simulink model "Solar_Seguidor_V2"  (R2021b)
settings: Solver=ode1  StartTime=0.0  StopTime=10  FixedStep=25e-6  RelTol=1e-3
PostLoadFcn:
  | %clc; clear all; close all;
  | %%%%%%%%%%%%%%%%%%%%%%%%%%%%%%%%%%%%%%%%%%%%%%%%
  | %%%%%%%%% Solar seguidor de rede %%%%%%%%%%
  | %%%%%%%%%%%%%%%%%%%%%%%%%%%%%%%%%%%%%%%%%%%%%%%%
  | %%%% Nominal Parameters %%%%
  | Pnom = 16e3;                                         % Potencia Nominal
  | Vnom_rms = 210;                                    % V linha rms
  | Vnom_peak = sqrt(2/3)*Vnom_rms;                     % V fase pico
  | FP_min = 1;                                       % Para suporte de reativo
  | Snom = Pnom/FP_min;                                 % Potencia aparente
  | Irms = Pnom/(sqrt(3)*Vnom_rms);                     % Ig rms
  | Inom_peak = Irms*sqrt(2);                           % Ig pico
  | Zbase = Vnom_peak/Inom_peak;                        % Impedancia Base
  | f = 60;                                             % Freq nominal
  | wnom = 2*pi*60;                                     % Freq Ang. nominal
  | m = 0.805;                                            % Indice mod nominal
  | Vdc = 2*(Vnom_peak/m);                              % Vcc
  | Vdc_2 = Vdc/2;                                      % Metade Vcc
  | Kconv = Zbase;                                      % Ganho conversor
  | %%%% Transformer %%%%
  | S_trafo = 250e3;                                      % transformer apparent power
  | Vrms_high = 400;                                   % transformer secondary voltage - Wye connection
  | Vrms_low = 210;                                   % transformer primary voltage - Delta connection
  | N = Vrms_high/Vrms_low;                             % transformation relationship
  | X_pu_trafo = 0.03;                                 % transformer p.u. reactance
  | Zb_trafo_high = ((Vrms_high)^2)/S_trafo;            % secondary base impedance
  | Zb_trafo = ((Vnom_rms)^2)/S_trafo;                  % primary base impedance
  | L_trafo = (X_pu_trafo*Zb_trafo)/wnom;               % primary inductance
  | %%%% LCL Filter Project %%%%
  | fsw = 105*60;%105*60;                                         % switching frequency
  | ripple = 0.05;                                       % current ripple
  | L1 = Vdc/(6*ripple*Inom_peak*fsw);                  % inductor L1
  |  RL1 = 0.005;                                        % L1 resistance
  |  Cbase = 1/(wnom*Kconv);                             % base capacitance
  |  Cf = 0.05*Cbase;                                    % filter capacitor
  | % Calculo do filtro
  | Sbase = 16e3;
  | %Sbase = 200e3*1.12;
  | V_LL = 210;
  | V_LG = 210/sqrt(3);
  | Vbase = V_LG*sqrt(2);
  | Ibase = (Sbase*sqrt(2))/(V_LG*3)*sqrt(3/2);
  | Zbase = (V_LL^2)/Sbase;
  | Rbase = Zbase;
  | Xbase = Zbase;
  | Lbase = Xbase/(2*pi*60);
  | Cbase = 1/(Xbase*2*pi*60);
  | w = 2*pi*60;
  | Q = 70;
  | Lf = 0.15*Lbase;
  | Cf = 0.05*Cbase;
  | fc = 1/(2*pi*sqrt(Lf*Cf));
  | R = (w*Lf)/Q;
  | Lf = L1;
  | R = RL1;
  | ka=0.2;                                             % attenuation factor
  | L2 = (sqrt(1/(ka^2))+1)/(Cf*((2*pi*fsw)^2));        % inductor L2
  | RL2 = 0.005;                                        % L2 resistance
  | w_res = sqrt((L1+L2+L_trafo)/(L1*L2*Cf));           % resonant angular frequency
  | f_res = w_res/(2*pi);                               % resonant frequency
  | Rf = 1/(3*w_res*Cf);                                % filter capacitor resistance
  | %%%%%%%%%%%%%%%%%%%%%%%%
  | %%%% Control Design %%%%
  | %%%%%%%%%%%%%%%%%%%%%%%%
  | %%%% Power Control %%%%
  | Ron = 0.0001;
  | tau_i = 0.5e-3;                                       % tempo de resposta
  | kp_current = (Lf+L_trafo)/tau_i;
  | ki_current = (R+Ron)/tau_i;
  | decouple = (wnom*Lf);
  | kp_current_pu = kp_current/Kconv;                  % Adaptando para pu
  | ki_current_pu = ki_current/Kconv;
  | decouple_pu = (wnom*Lf+(R+Ron))/Kconv;
  | %%%% Dc Link Control %%%%
  | Iext = Pnom/Vdc;
  | Kcc = Vdc/Iext;
  | Sbase = 16e3;
  | C_cc_proj = (Sbase/(2*pi*60*Vdc*Vdc*0.05));
  | 
  | % Controle de tensao
  | a = 3;
  | kp_dc = (C_cc_proj)/(2*a*tau_i);
  | ti_dc = (a^2)*tau_i;
  | ki_dc = kp_dc/ti_dc;
  | kp_dc_pu = (Kcc*C_cc_proj)/(2*a*tau_i);
  | ki_dc_pu = kp_dc_pu/ti_dc;
  | 
  | Ts =25e-6;
  | 
  | 
  |  Ts_Control=2*Ts;Ts_Power=Ts;
InitFcn:
  | %clc; clear all; close all;
  | %%%%%%%%%%%%%%%%%%%%%%%%%%%%%%%%%%%%%%%%%%%%%%%%
  | %%%%%%%%% Solar seguidor de rede %%%%%%%%%%
  | %%%%%%%%%%%%%%%%%%%%%%%%%%%%%%%%%%%%%%%%%%%%%%%%
  | %%%% Nominal Parameters %%%%
  | Pnom = 16e3;                                         % Potencia Nominal
  | Vnom_rms = 210;                                    % V linha rms
  | Vnom_peak = sqrt(2/3)*Vnom_rms;                     % V fase pico
  | FP_min = 1;                                       % Para suporte de reativo
  | Snom = Pnom/FP_min;                                 % Potencia aparente
  | Irms = Pnom/(sqrt(3)*Vnom_rms);                     % Ig rms
  | Inom_peak = Irms*sqrt(2);                           % Ig pico
  | Zbase = Vnom_peak/Inom_peak;                        % Impedancia Base
  | f = 60;                                             % Freq nominal
  | wnom = 2*pi*60;                                     % Freq Ang. nominal
  | m = 0.805;                                            % Indice mod nominal
  | Vdc = 2*(Vnom_peak/m);                              % Vcc
  | Vdc_2 = Vdc/2;                                      % Metade Vcc
  | Kconv = Zbase;                                      % Ganho conversor
  | %%%% Transformer %%%%
  | S_trafo = 250e3;                                      % transformer apparent power
  | Vrms_high = 400;                                   % transformer secondary voltage - Wye connection
  | Vrms_low = 210;                                   % transformer primary voltage - Delta connection
  | N = Vrms_high/Vrms_low;                             % transformation relationship
  | X_pu_trafo = 0.03;                                 % transformer p.u. reactance
  | Zb_trafo_high = ((Vrms_high)^2)/S_trafo;            % secondary base impedance
  | Zb_trafo = ((Vnom_rms)^2)/S_trafo;                  % primary base impedance
  | L_trafo = (X_pu_trafo*Zb_trafo)/wnom;               % primary inductance
  | %%%% LCL Filter Project %%%%
  | fsw = 105*60;%105*60;                                         % switching frequency
  | ripple = 0.05;                                       % current ripple
  | L1 = Vdc/(6*ripple*Inom_peak*fsw);                  % inductor L1
  |  RL1 = 0.005;                                        % L1 resistance
  |  Cbase = 1/(wnom*Kconv);                             % base capacitance
  |  Cf = 0.05*Cbase;                                    % filter capacitor
  | % Calculo do filtro
  | Sbase = 16e3;
  | %Sbase = 200e3*1.12;
  | V_LL = 210;
  | V_LG = 210/sqrt(3);
  | Vbase = V_LG*sqrt(2);
  | Ibase = (Sbase*sqrt(2))/(V_LG*3)*sqrt(3/2);
  | Zbase = (V_LL^2)/Sbase;
  | Rbase = Zbase;
  | Xbase = Zbase;
  | Lbase = Xbase/(2*pi*60);
  | Cbase = 1/(Xbase*2*pi*60);
  | w = 2*pi*60;
  | Q = 70;
  | Lf = 0.15*Lbase;
  | Cf = 0.05*Cbase;
  | fc = 1/(2*pi*sqrt(Lf*Cf));
  | R = (w*Lf)/Q;
  | Lf = L1;
  | R = RL1;
  | ka=0.2;                                             % attenuation factor
  | L2 = (sqrt(1/(ka^2))+1)/(Cf*((2*pi*fsw)^2));        % inductor L2
  | RL2 = 0.005;                                        % L2 resistance
  | w_res = sqrt((L1+L2+L_trafo)/(L1*L2*Cf));           % resonant angular frequency
  | f_res = w_res/(2*pi);                               % resonant frequency
  | Rf = 1/(3*w_res*Cf);                                % filter capacitor resistance
  | %%%%%%%%%%%%%%%%%%%%%%%%
  | %%%% Control Design %%%%
  | %%%%%%%%%%%%%%%%%%%%%%%%
  | %%%% Power Control %%%%
  | Ron = 0.0001;
  | tau_i = 0.5e-3;                                       % tempo de resposta
  | kp_current = (Lf+L_trafo)/tau_i;
  | ki_current = (R+Ron)/tau_i;
  | decouple = (wnom*Lf);
  | kp_current_pu = kp_current/Kconv;                  % Adaptando para pu
  | ki_current_pu = ki_current/Kconv;
  | decouple_pu = (wnom*Lf+(R+Ron))/Kconv;
  | %%%% Dc Link Control %%%%
  | Iext = Pnom/Vdc;
  | Kcc = Vdc/Iext;
  | Sbase = 16e3;
  | C_cc_proj = (Sbase/(2*pi*60*Vdc*Vdc*0.05));
  | 
  | % Controle de tensao
  | a = 3;
  | kp_dc = (C_cc_proj)/(2*a*tau_i);
  | ti_dc = (a^2)*tau_i;
  | ki_dc = kp_dc/ti_dc;
  | kp_dc_pu = (Kcc*C_cc_proj)/(2*a*tau_i);
  | ki_dc_pu = kp_dc_pu/ti_dc;
  | 
  | Ts =25e-6;
  | 
  | 
  |  Ts_Control=2*Ts;Ts_Power=Ts;
undefined symbols (not defined in the file): D1, Delta, DERS_models, DiscIntNeverNeededParam, eHS, I, Ia_PV, Ib_PV, Ic_PV, Left, parameter_set_id, ph, PV_system, type, V, Va_grid, Vb_grid, Vc_grid
libraries: powerlib_meascontrol x17, rtlab x14, spsThreePhaseSeriesRLCBranchLib x9, spsCurrentMeasurementLib x9, artemis x7, spsThreePhaseVIMeasurementLib x6, slpidlib x6, rteventslib x6, spsabctodq0Lib x4, spsThreePhaseTransformerTwoWindingsLib x3, simulink x3, spsPVArrayLib x3
(part 1 of 4)
settings Model: ARTEMISmethode_block_infos=$$__separator__$$Solar_Seguidor_V2/ARTEMIS Guide1$$__separator__$$  Creator=Lafae  LastModifiedBy=lafae
settings SolverCC: AlgebraicLoopSolver=LineSearch
settings DataIOCC: SaveOutput=off  SaveTime=off  ReturnWorkspaceOutputs=off
settings OptimizationCC: BlockReduction=off  OptimizeBlockIOStorage=off  BufferReuse=off  GlobalBufferReuse=off  ExpressionFolding=off  LocalBlockOutputs=off  OptimizeDataStoreBuffers=off  BusAssignmentInplaceUpdate=off
settings DebuggingCC: AlgebraicLoopMsg=none  MaxConsecutiveZCsMsg=none  MultiTaskDSMMsg=warning  ParameterOverflowMsg=warning  ModelReferenceExtraNoncontSigs=none  SFMachineParentedDataDiag=warning  ArithmeticOperatorsInVariantConditions=warning
settings SFSimCC: CustomCodeUndefinedFunction=UseInterfaceOnly

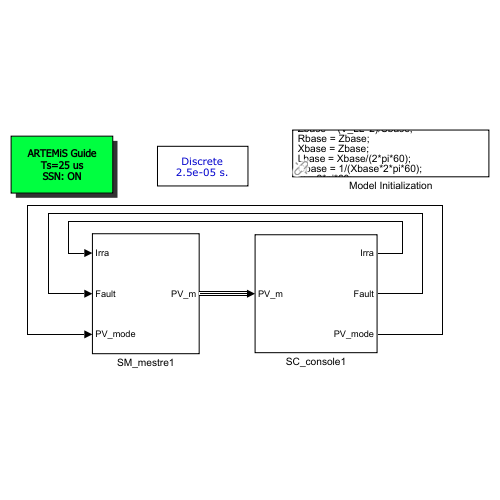
[thumbnail: Simulink's stored preview of the top-level diagram]
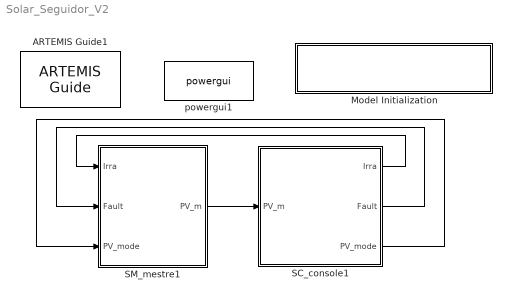
== system Solar_Seguidor_V2 ==
  ARTEMIS Guide1 : artemis/ARTEMIS/ARTEMIS Guide  Tag=art7.5  Description=New ARTEMiS block v 7.5b (R2015b+)  lock=on  Ts=Ts  ssn=on  opt=art5  dyna=off  nb_perm=4  RT_fullcomp=off  ssn_itvc=off  ssn_ivic=off  ssn_ext=off  ssn_solver=Art5  iter_type=iSWITCH and iMOV only (default)  ssn_ImpulseLoopBlockedStateUpdate=5  ssn_mov_iter_number=5  ssn_switch_iter_number=3  ssn_lu_or_ldlt=LU (more robust)  ssn_nib_type_verify=on  ssn_use_lu=on  ssn_use_ldlt=off  ssn_impulse=on  ssn_quasimpulse=off  ssn_impulse_loop=5  paraExtinctionThy=off  Thy_Impulse=on  dtc=Off  dtc_opt=normal  ao=off  simtype=off  ct_mac=off  lin_mov=off  lsp=[0.001 2]  spike_skip=Disabled  dtc_extra=1  dtc_sws=normal  dtc_pied=0.5  SPSRulesBlock=SPSRules  tre=off  ctmm=off  LF=off  dpl_type=ARTEMiS DPL  rlc_type=off  custom_type=off  para=on  ssn_full_iteration=off  ssn_init_cond=block only
  Model Initialization : Subsystem  AncestorBlock=artemis/Tools /Misc/Model Initialization  mask(Model Functions){InitFcnX=|, prel=off, posl=on, inif=on, strf=off}
      mask InitFcnX=|
      | %clc; clear all; close all;
      | %%%%%%%%%%%%%%%%%%%%%%%%%%%%%%%%%%%%%%%%%%%%%%%%
      | %%%%%%%%% Solar seguidor de rede %%%%%%%%%%
      | %%%%%%%%%%%%%%%%%%%%%%%%%%%%%%%%%%%%%%%%%%%%%%%%
      | %%%% Nominal Parameters %%%%
      | Pnom = 16e3;                                         % Potencia Nominal
      | Vnom_rms = 210;                                    % V linha rms
      | Vnom_peak = sqrt(2/3)*Vnom_rms;                     % V fase pico
      | FP_min = 1;                                       % Para suporte de reativo
      | Snom = Pnom/FP_min;                                 % Potencia aparente
      | Irms = Pnom/(sqrt(3)*Vnom_rms);                     % Ig rms
      | Inom_peak = Irms*sqrt(2);                           % Ig pico
      | Zbase = Vnom_peak/Inom_peak;                        % Impedancia Base
      | f = 60;                                             % Freq nominal
      | wnom = 2*pi*60;                                     % Freq Ang. nominal
      | m = 0.805;                                            % Indice mod nominal
      | Vdc = 2*(Vnom_peak/m);                              % Vcc
      | Vdc_2 = Vdc/2;                                      % Metade Vcc
      | Kconv = Zbase;                                      % Ganho conversor
      | %%%% Transformer %%%%
      | S_trafo = 250e3;                                      % transformer apparent power
      | Vrms_high = 400;                                   % transformer secondary voltage - Wye connection
      | Vrms_low = 210;                                   % transformer primary voltage - Delta connection
      | N = Vrms_high/Vrms_low;                             % transformation relationship
      | X_pu_trafo = 0.03;                                 % transformer p.u. reactance
      | Zb_trafo_high = ((Vrms_high)^2)/S_trafo;            % secondary base impedance
      | Zb_trafo = ((Vnom_rms)^2)/S_trafo;                  % primary base impedance
      | L_trafo = (X_pu_trafo*Zb_trafo)/wnom;               % primary inductance
      | %%%% LCL Filter Project %%%%
      | fsw = 105*60;%105*60;                                         % switching frequency
      | ripple = 0.05;                                       % current ripple
      | L1 = Vdc/(6*ripple*Inom_peak*fsw);                  % inductor L1
      |  RL1 = 0.005;                                        % L1 resistance
      |  Cbase = 1/(wnom*Kconv);                             % base capacitance
      |  Cf = 0.05*Cbase;                                    % filter capacitor
      | % Calculo do filtro
      | Sbase = 16e3;
      | %Sbase = 200e3*1.12;
      | V_LL = 210;
      | V_LG = 210/sqrt(3);
      | Vbase = V_LG*sqrt(2);
      | Ibase = (Sbase*sqrt(2))/(V_LG*3)*sqrt(3/2);
      | Zbase = (V_LL^2)/Sbase;
      | Rbase = Zbase;
      | Xbase = Zbase;
      | Lbase = Xbase/(2*pi*60);
      | Cbase = 1/(Xbase*2*pi*60);
      | w = 2*pi*60;
      | Q = 70;
      | Lf = 0.15*Lbase;
      | Cf = 0.05*Cbase;
      | fc = 1/(2*pi*sqrt(Lf*Cf));
      | R = (w*Lf)/Q;
      | Lf = L1;
      | R = RL1;
      | ka=0.2;                                             % attenuation factor
      | L2 = (sqrt(1/(ka^2))+1)/(Cf*((2*pi*fsw)^2));        % inductor L2
      | RL2 = 0.005;                                        % L2 resistance
      | w_res = sqrt((L1+L2+L_trafo)/(L1*L2*Cf));           % resonant angular frequency
      | f_res = w_res/(2*pi);                               % resonant frequency
      | Rf = 1/(3*w_res*Cf);                                % filter capacitor resistance
      | %%%%%%%%%%%%%%%%%%%%%%%%
      | %%%% Control Design %%%%
      | %%%%%%%%%%%%%%%%%%%%%%%%
      | %%%% Power Control %%%%
      | Ron = 0.0001;
      | tau_i = 0.5e-3;                                       % tempo de resposta
      | kp_current = (Lf+L_trafo)/tau_i;
      | ki_current = (R+Ron)/tau_i;
      | decouple = (wnom*Lf);
      | kp_current_pu = kp_current/Kconv;                  % Adaptando para pu
      | ki_current_pu = ki_current/Kconv;
      | decouple_pu = (wnom*Lf+(R+Ron))/Kconv;
      | %%%% Dc Link Control %%%%
      | Iext = Pnom/Vdc;
      | Kcc = Vdc/Iext;
      | Sbase = 16e3;
      | C_cc_proj = (Sbase/(2*pi*60*Vdc*Vdc*0.05));
      |
      | % Controle de tensao
      | a = 3;
      | kp_dc = (C_cc_proj)/(2*a*tau_i);
      | ti_dc = (a^2)*tau_i;
      | ki_dc = kp_dc/ti_dc;
      | kp_dc_pu = (Kcc*C_cc_proj)/(2*a*tau_i);
      | ki_dc_pu = kp_dc_pu/ti_dc;
      |
      | Ts =25e-6;
      |
      |
      |  Ts_Control=2*Ts;Ts_Power=Ts;
      mask prompts: InitFcnX "Initialisation"; prel "Preload Function"; posl "PostLoad Function"; inif "InitFcn"; strf "StartFcn"
      mask init:
      | currentBlock = gcb;
      | root = bdroot(currentBlock);
      | 
      | if ~strcmp(get_param(root,'BlockDiagramType'),'library')
      |     if prel==1
      |         set_param(root, 'PreLoadFcn', InitFcnX);
      |     else
      |         set_param(root, 'PreLoadFcn', '');
      |     end
      |     if inif==1
      |         set_param(root, 'InitFcn', InitFcnX);
      |     else
      |         set_param(root, 'InitFcn', '');
      |     end
      |     if strf==1
      |         set_param(root, 'StartFcn', InitFcnX);
      |     else
      |         set_param(root, 'StartFcn', '');
      |     end
      |     if posl==1
      |         set_param(root, 'PostLoadFcn', InitFcnX);
      |     else
      |         set_param(root, 'PostLoadFcn', '');
      |     end
      | end
      | 
      | pos = get_param(currentBlock, 'Position');
      | width = pos(3) - pos(1); height = pos(4) - pos(2);
      | txt = [ upper(root) '\n' '- InitFcn. . . . . '  get_param(root, 'InitFcn') ];
      settings: CopyFcn=set_param(gcb,'LinkStatus','inactive')
      mask Display: text(5, height*0.5, txt, 'horizontalAlignment', 'left', 'verticalAlignment', 'middle') ;
  SC_console1 : Subsystem
  SM_mestre1 : Subsystem
  powergui1 : spspowerguiLib/powergui  Priority=1  SimulationMode=Discrete  SampleTime=Ts  frequency=60  Iterations=50  frequencyindice=0  Pbase=100e6  ErrMax=1e-4  UnitsV=kV  UnitsW=MW  buscounter=0  FunctionMessages=off  echomessages=off  EnableUseOfTLC=off  CurrentSourceSwitches=off  DisableSnubberDevices=off  DisableRonSwitches=off  DisableVfSwitches=off  DisplayEquations=off  AutomaticDiscreteSolvers=off  SolverType=Tustin/Backward Euler (TBE)  Interpol=off  ExternalGateDelay=off  methode=off  Ts=0  x0status=blocks  SPID=off  SwTol=0  HookPort=off  NonlinearTolerance=0  nMaxIteration=15  ContinueOnMaxIteration=off  RestoreLinks=warning  ResistiveCurrentMeasurement=off  Frange=[0:2:500]  Ylog=off  Xlog=on  ShowGrid=off  save=off  variable=ZData  structure=0  ZoomFFT=on  StartTime=0.0  cycles=1  DisplayStyle=1  fundamental=60  FreqAxis=off  MaxFrequency=1000  frequencyindicesteady=1  RmsSteady=1  display=off
  wires:
  SM_mestre1/1(PV_m) -> SC_console1/1(PV_m)
  SC_console1/3(PV_mode) -> SM_mestre1/3(PV_mode)
  SC_console1/2(Fault) -> SM_mestre1/2(Fault)
  SC_console1/1(Irra) -> SM_mestre1/1(Irra)

== system Solar_Seguidor_V2/Model Initialization ==

== system Solar_Seguidor_V2/SC_console1 ==
  note: Fault:
      | 0: Off
      | 1: On
  PV_m : Inport
  Bus Selector : BusSelector  OutputSignals=THD_Ia,Iabc_PV_pu,Iabc_grid_pu,Vdc,P_PV,Freq
  Command Fault (From 0 To 1) : ManualSwitch  CurrentSetting=0
  Constant : Constant  Value=500
  Constant1 : Constant
  Currents_AC : Scope  NumInputPorts=2
  Display : Display
  Fault_Subsystem : Subsystem
  Frequence : Scope
  OpComm : rtlab/OpComm  nbport=1  groupe_acq=1  subsys_rate=0  st=0  Synchronization=on  Interpolation=on  Threshold=1.0  Missed_Data=off  Sim_Time=off  Samples=off  dynSigOut=off  from_console=0  warning_done=off  writeOpCommFile=off  Offset=off
      settings: SourceProductName=RT-LAB
  Power_DC : Scope
  Scope : Scope
  Stair Generator1 : spsStairGeneratorLib/Stair Generator  Commented=on  t=[0, 1, 3, 5,7]  e=[10, 4, 7.5, 10,2.5]*1e2  Ts=0
  THD : Scope
  Vdc_m : Scope
  c1 : Constant
  c3 : Constant  Value=0
  Irra : Outport
  Fault : Outport  Port=2
  PV_mode : Outport  Port=3
  wires:
  [Iabc_PV] -> Currents_AC/1
  [Iabc_grid] -> Currents_AC/2
  PV_m/1 -> OpComm/1
  Bus Selector/2 -> [Iabc_PV]  "<Iabc_PV_pu>"
  Constant/1 -> Irra/1
  Fault_Subsystem/1(Out1) -> Fault/1
  c1/1 -> Command Fault (From 0 To 1)/1
  c3/1 -> Command Fault (From 0 To 1)/2
  Command Fault (From 0 To 1)/1 -> Fault_Subsystem/1(cmd)
  Constant1/1 -> PV_mode/1
  [Iabc_PV] -> Scope/1
  OpComm/1 -> Bus Selector/1
  Bus Selector/1 -> THD/1  "<THD_Ia>"
  Bus Selector/3 -> [Iabc_grid]  "<Iabc_grid_pu>"
  Bus Selector/4 -> Vdc_m/1  "<Vdc>"
  Bus Selector/5 -> Display/1, Power_DC/1  "<P_PV>"
  Bus Selector/6 -> Frequence/1  "<Freq>"

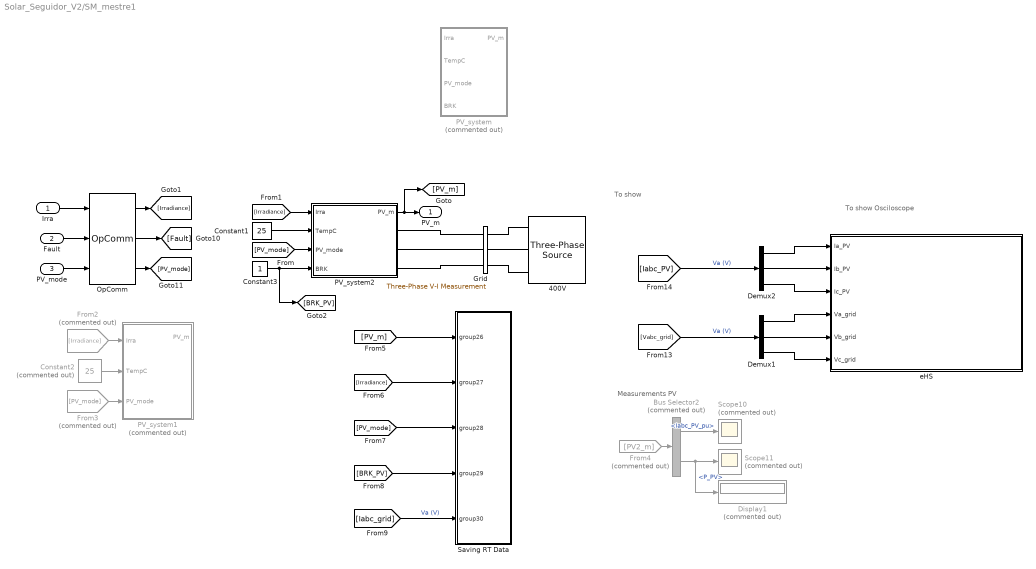
== system Solar_Seguidor_V2/SM_mestre1 ==
  note: To show Osciloscope
  note: To show
  note: Measurements PV
  Irra : Inport
  Fault : Inport  Port=2
  PV_mode : Inport  Port=3
  "400V " : spsThreePhaseSourceLib/Three-Phase Source  InternalConnection=Yg  VoltagePhases=off  Voltage=400  PhaseAngle=0  Voltage_phases=[25e3 25e3 25e3]/sqrt(3)  PhaseAngles_phases=[0 -120 +120]  Frequency=60  NonIdealSource=on  SpecifyImpedance=on  Resistance=0.8929  Inductance=16.58e-3  ShortCircuitLevel=2500e6  BaseVoltage=400  XRratio=7  BusType=swing  Pref=0  Qref=0  Prefabc=[10e3, 10e3, 10e3]  Qrefabc=[0, 0, 0]  Qmin=-inf  Qmax=inf
  Bus Selector2 : BusSelector  Commented=on  OutputSignals=Iabc_PV_pu,P_PV
  Constant1 : Constant  Value=25
  Constant2 : Constant  Commented=on  Value=25
  Constant3 : Constant
  Demux1 : Demux  Outputs=3
  Demux2 : Demux  Outputs=3
  Display1 : Display  Commented=on
  From2 : From  Commented=on  GotoTag=Irradiance
  From3 : From  Commented=on  GotoTag=PV_mode
  From4 : From  Commented=on  GotoTag=PV2_m
  Grid : spsThreePhaseVIMeasurementLib/Three-Phase V-I Measurement  VoltageMeasurement=phase-to-ground  SetLabelV=on  LabelV=Vabc_grid  Vpu=off  VpuLL=off  CurrentMeasurement=yes  SetLabelI=on  LabelI=Iabc_grid  Ipu=off  Pbase=100e6  Vbase=500e3  OutputType=Complex  PhasorSimulation=off  PSBequivalent=0
  OpComm : rtlab/OpComm  nbport=3  groupe_acq=1  subsys_rate=0  st=0  Synchronization=on  Interpolation=on  Threshold=1.0  Missed_Data=off  Sim_Time=off  Samples=off  dynSigOut=off  from_console=1  warning_done=off  writeOpCommFile=off  Offset=off
      settings: SourceProductName=RT-LAB
  PV_system : Subsystem  Commented=on  mask(PV system){Q=0.25, Iq_ref=0.25, Kp_dc=kp_dc_pu, Ki_dc=ki_dc_pu, Kp_i=kp_current_pu, Ki_i=ki_current_pu}
      mask prompts: Q "Active Power"; Iq_ref "Reactive Power"; Kp_dc "Proportional Gain"; Ki_dc "Integral Gain"; Kp_i "Proportional Gain"; Ki_i "Integral Gain"
      mask help: This is a example of a PV system
      mask Help: This is a example of a PV system
      mask DialogControl Container5 Prompt: Controllers
      mask DialogControl Container6 Prompt: DC Link
      mask DialogControl Container7 Prompt: Current Controller
      mask Display:
      | %image('$imagefile'); % Use "Edit Image" on toolstrip to change.
      | 
      | port_label('input',1,'Irr')
      | port_label('input',2,'Temp')
      | port_label('input',3,'PV Mode')
      | port_label('input',4,'BRK')
      | 
      | 
      | %output
      | port_label('output',1,'PV_m')
      | 
      | %electrical
      | port_label('Rconn',1,'Va')
      | port_label('Rconn',2,'Vb')
      | port_label('Rconn',3,'Vc')
  PV_system1 : Subsystem  Commented=on  AncestorBlock=DERS_models/PV_system  mask(PV system){Q=0.25, Iq_ref=0.25, Kp_dc=kp_dc_pu, Ki_dc=ki_dc_pu, Kp_i=kp_current_pu, Ki_i=ki_current_pu}
      mask prompts: Q "Active Power"; Iq_ref "Reactive Power"; Kp_dc "Proportional Gain"; Ki_dc "Integral Gain"; Kp_i "Proportional Gain"; Ki_i "Integral Gain"
      mask help: This is a example of a PV system
      mask Help: This is a example of a PV system
      mask DialogControl Container5 Prompt: Controllers
      mask DialogControl Container6 Prompt: DC Link
      mask DialogControl Container7 Prompt: Current Controller
      mask Display:
      | %image('$imagefile'); % Use "Edit Image" on toolstrip to change.
      | 
      | port_label('input',1,'Irr')
      | port_label('input',2,'Temp')
      | port_label('input',3,'PV Mode')
      | %port_label('input',4,'BRK')
      | 
      | 
      | %output
      | port_label('output',1,'PV_m')
      | 
      | %electrical
      | port_label('Rconn',1,'Va')
      | port_label('Rconn',2,'Vb')
      | port_label('Rconn',3,'Vc')
  PV_system2 : Subsystem  AncestorBlock=DERS_models/PV_system  mask(PV system){Q=1, Iq_ref=0, Kp_dc=kp_dc_pu, Ki_dc=ki_dc_pu, Kp_i=kp_current_pu, Ki_i=ki_current_pu}
      mask prompts: Q "Active Power"; Iq_ref "Reactive Power"; Kp_dc "Proportional Gain"; Ki_dc "Integral Gain"; Kp_i "Proportional Gain"; Ki_i "Integral Gain"
      mask help: This is a example of a PV system
      mask Help: This is a example of a PV system
      mask DialogControl Container5 Prompt: Controllers
      mask DialogControl Container6 Prompt: DC Link
      mask DialogControl Container7 Prompt: Current Controller
      mask Display:
      | image('$imagefile'); % Use "Edit Image" on toolstrip to change.
      | 
      | 
      | port_label('input',1,'Irr')
      | port_label('input',2,'Temp')
      | port_label('input',3,'PV Mode')
      | %port_label('input',4,'BRK')
      | 
      | 
      | %output
      | port_label('output',1,'PV_m')
      | 
      | %electrical
      | port_label('Rconn',1,'Va')
      | port_label('Rconn',2,'Vb')
      | port_label('Rconn',3,'Vc')
  Saving RT Data : Subsystem  mask{Ts=Ts, Decimation26=3, varname26=PV, Filename26=PV_m.mat, nls26=38, ld26=40, Decimation27=3, varname27=Irra, Filename27=Irradiance.mat, nls27=15, ld27=40, Decimation28=3, varname28=PV_mode, Filename28=PV_mode.mat, nls28=19, ld28=40, Decimation29=3, varname29=BRK_PV, Filename29=BRK_PV.mat, nls29=19, ld29=40, Decimation30=3, varname30=Iabc_grid, Filename30=Iabc_grid.mat, nls30=20, ld30=40}
      mask prompts: Ts "Ts (s)"; Decimation26 "Decimation factor"; varname26 "Variable name"; Filename26 "FileName"; nls26 "Number of logged signals"; ld26 "Logging duration (s)"; Decimation27 "Decimation factor"; varname27 "Variable name"; Filename27 "FileName"; nls27 "Number of logged signals"; ld27 "Logging duration (s)"; Decimation28 "Decimation factor"; varname28 "Variable name"; Filename28 "FileName"; nls28 "Number of logged signals"; ld28 "Logging duration (s)"; Decimation29 "Decimation factor"; varname29 "Variable name"; Filename29 "FileName"; nls29 "Number of logged signals"; ld29 "Logging duration (s)"; Decimation30 "Decimation factor"; varname30 "Variable name"; Filename30 "FileName"; nls30 "Number of logged signals"; ld30 "Logging duration (s)"
      mask help: This block contains the 5 groups of OpWriteFile (26, 27, 28 29 and 30) blocks that write signals to a binary file (.mat), files that are in the binary data container format that MATLAB uses.
      mask TypeOptions Decimation26: OpWriteFile26/Decimation
      mask TypeOptions varname26: OpWriteFile26/varname
      mask TypeOptions Filename26: OpWriteFile26/Filename
      mask TypeOptions Decimation27: OpWriteFile27/Decimation
      mask TypeOptions varname27: OpWriteFile27/varname
      mask TypeOptions Filename27: OpWriteFile27/Filename
      mask TypeOptions Decimation28: OpWriteFile28/Decimation
      mask TypeOptions varname28: OpWriteFile28/varname
      mask TypeOptions Filename28: OpWriteFile28/Filename
      mask TypeOptions Decimation29: OpWriteFile29/Decimation
      mask TypeOptions varname29: OpWriteFile29/varname
      mask TypeOptions Filename29: OpWriteFile29/Filename
      mask TypeOptions Decimation30: OpWriteFile30/Decimation
      mask TypeOptions varname30: OpWriteFile30/varname
      mask TypeOptions Filename30: OpWriteFile30/Filename
      mask DialogControl DescGroupVar Prompt: Saving RT Data
      mask DialogControl Container4 Prompt: Group 26
      mask DialogControl Container9 Prompt: Group 27
      mask DialogControl Container10 Prompt: Group 28
      mask DialogControl Container11 Prompt: Group 29
      mask DialogControl Container12 Prompt: Group 30
  Scope10 : Scope  Commented=on
  Scope11 : Scope  Commented=on
  eHS : Subsystem  mask{ModelsList=<No circuit selected>, Timestamp=Unable to import previously loaded circuit, ShowInLibBrowser=on, SourceSetList=Internal, ActiveSetList=(0) Default set}
      mask help:
      | This block allows the configuration and the control of an FPGA-based circuit simulation using eHS Power Electronics toolbox.
      | The circuit is edited using OPAL-RT Schematic Editor.
      settings: CopyFcn=set_param(gcb,'LinkStatus','none');  OpenFcn=ehsGen4BlockLastModelLoadedCb(gcb)
      mask Help: web(['file:///' getenv('EFPGASIM_ROOT') '/Docs/html/eFPGAsim/efs_eHSgen4_SE.html']);
      mask TypeOptions ModelsList: <No circuit selected>
      mask Callback ModelsList: ehsGen4BlockFillModelListCb(gcb);
      mask TypeOptions SourceSetList: Internal | External
      mask Callback SourceSetList: ehsGen4BlockParamSetSourceCb(gcb);
      mask TypeOptions ActiveSetList: (0) Default set
      mask DialogControl ParameterGroupVar Prompt: Circuit
      mask DialogControl ModelName Prompt: Name
      mask DialogControl Refresh Callback: ehsGen4BlockFillModelListCb(gcb);
      mask DialogControl Edit Prompt: Edit
      mask DialogControl Edit Callback: ehsGen4BlockEditModelCb(gcb);
      mask DialogControl CreateNew Prompt: Create new
      mask DialogControl CreateNew Callback: ehsGen4BlockCreateModelCb(gcb);
      mask DialogControl Load Prompt: Load circuit
      mask DialogControl Load Callback: ehsGen4BlockLoadModelCb(gcb);
      mask DialogControl ErrorLink Prompt: More configuration details
      mask DialogControl ErrorLink Callback: ehsGen4BlockNotificationPopupCb(gcb);
      mask DialogControl ParameterSetGroup Prompt: Parameter set
      mask DialogControl Source Prompt: Source
      mask DialogControl ActiveSet Prompt: Active set
      mask DialogControl Uuid Prompt: 2fa47343-3408-4814-9c5b-84dec2eff337
      mask DialogControl LastModelLoaded Prompt: Test_IO - v1
      mask Display:
      | fprintf('eHS\n\n')
      | fprintf(ehsGen4BlockGetLastModelLoaded(gcb))
      | ehsGen4BlockUpdateConstantBlockCb(gcb)
      | ehsGen4BlockAddLabel
  PV_m : Outport
  wires:
  Demux2/2 -> eHS/2(Ib_PV)
  Demux1/2 -> eHS/5(Vb_grid)
  Demux2/1 -> eHS/1(Ia_PV)
  Demux1/3 -> eHS/6(Vc_grid)
  Demux1/1 -> eHS/4(Va_grid)
  [Iabc_PV] -> Demux2/1  "Va (V)"
  [Vabc_grid] -> Demux1/1  "Va (V)"
  Demux2/3 -> eHS/3(Ic_PV)
  Irra/1 -> OpComm/1
  Fault/1 -> OpComm/2
  OpComm/2 -> [Fault]
  PV_mode/1 -> OpComm/3
  OpComm/3 -> [PV_mode]
  Constant1/1 -> PV_system2/2(TempC)
  PV_system2/1(PV_m) -> [PV_m], PV_m/1
  [PV_mode] -> PV_system2/3(PV_mode)
  OpComm/1 -> [Irradiance]
  [Irradiance] -> PV_system2/1(Irra)
  From2/1 -> PV_system1/1(Irra)
  Constant2/1 -> PV_system1/2(TempC)
  From3/1 -> PV_system1/3(PV_mode)
  From4/1 -> Bus Selector2/1
  Bus Selector2/1 -> Scope10/1  "<Iabc_PV_pu>"
  Bus Selector2/2 -> Display1/1, Scope11/1  "<P_PV>"
  Constant3/1 -> [BRK_PV], PV_system2/4(BRK)
  [PV_m] -> Saving RT Data/1(group26)
  [Irradiance] -> Saving RT Data/2(group27)
  [PV_mode] -> Saving RT Data/3(group28)
  [BRK_PV] -> Saving RT Data/4(group29)
  [Iabc_grid] -> Saving RT Data/5(group30)  "Va (V)"
  connections:
  Grid/RConn2 -- PV_system2/RConn2
  PV_system2/RConn1 -- Grid/RConn1
  PV_system2/RConn3 -- Grid/RConn3
  "400V "/RConn2 -- Grid/LConn2
  "400V "/RConn1 -- Grid/LConn1
  "400V "/RConn3 -- Grid/LConn3

== system Solar_Seguidor_V2/SC_console1/Fault_Subsystem ==
  note: Note: This is the control of the three-phase fault.
  cmd : Inport
  Constant1 : Constant  Value=0
  On Delay : spsOnDelayLib/On Delay  DelayType=On delay  delay=5/60  ic=0  Ts=0
      settings: SourceProductBaseCode=PS
  Scope : Scope
  Switch : Switch  Criteria=u2 > Threshold
  Out1 : Outport
  wires:
  Switch/1 -> Scope/1, Out1/1
  Constant1/1 -> Switch/1
  On Delay/1 -> Switch/2
  cmd/1 -> Switch/3, On Delay/1

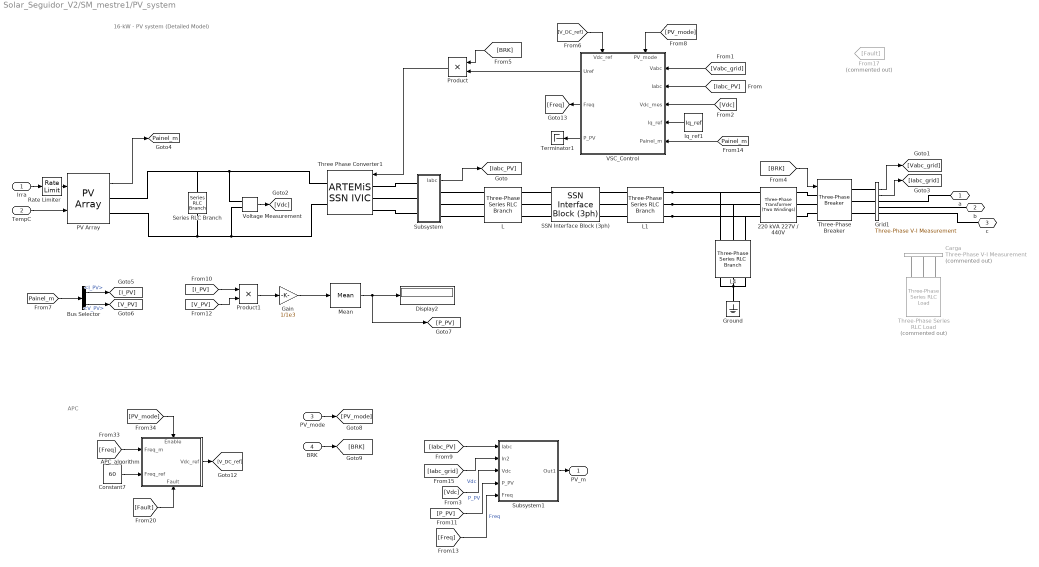
== system Solar_Seguidor_V2/SM_mestre1/PV_system ==
  note: 16-kW - PV system (Detailed Model)
  note: APC
  Irra : Inport
  TempC : Inport  Port=2
  PV_mode : Inport  Port=3
  BRK : Inport  Port=4
  220 kVA 227V / 440V : spsThreePhaseTransformerTwoWindingsLib/Three-Phase Transformer (Two Windings)  Winding1Connection=Yg  Winding2Connection=Delta (D1)  CoreType=Three single-phase transformers  SetSaturation=off  Hysteresis=off  DataFile='hysteresis'  SetInitialFlux=off  Measurements=None  UNITS=pu  NominalPower=[220e3 , 60 ]  Winding1=[400 , 0.001 , 0.03 ]  Winding2=[210 , 0.001 , 0.03 ]  Rm=500  Lm=500  L0=0.5  Saturation=[ 0,0 ; 0.0024,1.2 ; 1.0,1.52 ]  InitialFluxes=[ 0.8 , -0.8 , 0.7 ]  BreakLoop=off  DiscreteSolver=Trapezoidal iterative  DataType=off  TransfoNumber=0
  APC_algorithm : Subsystem
      settings: PortSchema="{\"entries\":[{\"content\":{\"sides\":[{\"content\":{\"connectorIds\":[\"In1\",\"In2\"]},\"type\":\"ConnectorPlacement.EquallySpacedRectSide\",\"uuid\":\"40656380-5e11-4201-a16e-0974ed2bdfa3\"},{\"content\":{\"connectorIds\":[\"Out1\"],\"side\":\"RIGHT\"},\"type\":\"ConnectorPlacement.EquallySpacedRectSide\",\"uuid\":\"b720f4a2-445d-4911-b95b-a16e7ba2ef90\"},{\"content\":{\"connectorIds\":[\"In3\"],\"side\":\"TOP\"},\"type\":\"ConnectorPlacement.EquallySpacedRectSide\",\"uuid\":\"61735eee-8c6f-4b86-833d-6912c6cea25a\"},{\"content\":{\"connectorIds\":[\"In4\"],\"side\":\"BOTTOM\"},\"type\":\"ConnectorPlacement.EquallySpacedRectSide\",\"uuid\":\"0dbf41d0-9732-4713-8148-d584ab86d8ba\"},{\"content\":{\"connectorIds\":[],\"side\":\"HIDDEN\"},\"type\":\"ConnectorPlacement.EquallySpacedRectSide\",\"uuid\":\"d2c68c6b-be31-4766-a941-11238d66741c\"}]},\"type\":\"ConnectorPlacement.EquallySpacedConnector\",\"uuid\":\"e0287d46-a6c7-46a5-bd63-f4e94fb98690\"}],\"packageUris\":[\"http://schema.mathworks.com/mf0/Connector/R2020b\"],\"version\":\"1.0\"}"
  Bus Selector : BusSelector  OutputSignals=I_PV,V_PV
  Carga : powerlib/Measurements/Three-Phase V-I Measurement  Commented=on  VoltageMeasurement=phase-to-ground  SetLabelV=on  LabelV=Vcarga  Vpu=off  VpuLL=off  CurrentMeasurement=yes  SetLabelI=on  LabelI=Icarga  Ipu=off  Pbase=100e6  Vbase=500e3  OutputType=Magnitude  PhasorSimulation=off  PSBequivalent=0
  Constant7 : Constant  Value=60
  Display2 : Display
  From17 : From  Commented=on  GotoTag=Fault
  Gain : Gain  Gain=1/1e3
  Grid1 : spsThreePhaseVIMeasurementLib/Three-Phase V-I Measurement  VoltageMeasurement=phase-to-ground  SetLabelV=off  LabelV=Vabc_grid  Vpu=off  VpuLL=off  CurrentMeasurement=yes  SetLabelI=off  LabelI=Iabc_grid  Ipu=off  Pbase=100e6  Vbase=500e3  OutputType=Magnitude  PhasorSimulation=off  PSBequivalent=0
  Ground : spsGroundLib/Ground  LConnTagsString=a
  Iq_ref1 : Constant  Value=Iq_ref
  L : spsThreePhaseSeriesRLCBranchLib/Three-Phase Series RLC Branch  LConnTagsString=A|B|C  RConnTagsString=A|B|C  BranchType=R  Resistance=R  Inductance=500e-6/2  Capacitance=inf  Measurements=None
  L1 : spsThreePhaseSeriesRLCBranchLib/Three-Phase Series RLC Branch  LConnTagsString=A|B|C  RConnTagsString=A|B|C  BranchType=L  Resistance=500e-6*377/50/2  Inductance=Lf  Capacitance=inf  Measurements=None
  L4 : spsThreePhaseSeriesRLCBranchLib/Three-Phase Series RLC Branch  LConnTagsString=A|B|C  RConnTagsString=A|B|C  BranchType=R  Resistance=1e8  Inductance=Lf  Capacitance=Cf  Measurements=None
  Mean : powerlib_meascontrol/Measurements/Mean  Freq=60  Vinit=0  Ts=0
  PV Array : spsPVArrayLib/PV Array  Npar=5  Nser=14  PlotType=array @ 1000 W/m2 & specified temperatures  S_vec=[ 1000]  Temp_C_vec=[ 25 ]  ModuleName=Trina Solar TSM-240PA05.30  PlotWhenSelected=off  Pm=239.856  Ncell=60  Voc=37.2  Isc=8.37  Vm=30.4  Im=7.89  beta_Voc_pc=-0.35  alpha_Isc_pc=0.06  beta_Voc=-0.1302  alpha_Isc=0.005022  IL=8.3942  I0=1.9964e-10  nI=0.98701  Rsh=355.1808  Rs=0.28785  RobustModel=off  RobustCellTemperature=313.3991  BAL=on  Tc=1e-6  Tfilter=5e-5
      settings: AttributesFormatString=|
      | %<ModuleName>
      | %<Nser>-module string
      | %<Npar> parallel strings
  Product : Product
  Product1 : Product
  Rate Limiter : RateLimiter  RisingSlewLimit=5000  FallingSlewLimit=-5000  SampleTimeMode=inherited  LinearizeAsGain=off
  SSN Interface Block (3ph) : artemis/SSN/Nodal Interface Blocks/SSN Interface Block (3ph)  nb_phase=3  nb_port=2  p1_type=I-type(Left)  p2_type=V-type (Right)  p3_type=V-type(Left)  p4_type=V-type(Left)  p5_type=V-type(Left)  p6_type=V-type(Left)  p7_type=V-type(Left)  p8_type=V-type(Left)  p9_type=V-type(Left)  p10_type=V-type(Left)  p11_type=V-type(Left)  p12_type=V-type(Left)  p13_type=V-type(Left)  p14_type=V-type(Left)  p15_type=V-type(Left)  p16_type=V-type(Left)  I_port_shunt_resistance=1e9
  Series RLC Branch : spsSeriesRLCBranchLib/Series RLC Branch  LConnTagsString=__new0  RConnTagsString=__new0  BranchType=C  Resistance=1  Inductance=1e-3  SetiL0=off  InitialCurrent=0  Capacitance=C_cc_proj  Setx0=on  InitialVoltage=Vdc  Measurements=None
  Subsystem : Subsystem
  Subsystem1 : Subsystem
  Terminator1 : Terminator
  Three Phase Converter1 : ssn_inverter_model/ARTEMiS SSN IVIC  Arms=3  SnubberResistance=800  SnubberCapacitance=inf  Device=IGBT / Diodes  Ron=Ron  Lon=0  ForwardVoltages=[0.001 0.001]  ForwardVoltage=0  GTOparameters=[ 10e-6 , 20e-6 ]  IGBTparameters=[ 1e-6 , 2e-6 ]*0  Measurements=None  Measurements_2=None  converterType=Rectifier
  Three-Phase Series RLC Load : powerlib/Elements/Three-Phase Series RLC Load  Commented=on  LConnTagsString=A|B|C  Configuration=Y (grounded)  NominalVoltage=227  Vabc=[1e3 1e3 1e3]  Vabcp=[1e3 1e3 1e3]  NominalFrequency=60  UnbalancedPower=off  ActivePower=80e3  InductivePower=15e3  CapacitivePower=0  Pabc=[10e3 9e3 11e3]  QLabc=[100 90 110]  QCabc=[100 90 110]  Pabcp=[10e3 9e3 11e3]  QLabcp=[100 90 110]  QCabcp=[100 90 110]  Measurements=None  LoadType=constant Z
  Three-Phase Breaker : spsThreePhaseBreakerLib/Three-Phase Breaker  InitialState=open  SwitchA=on  SwitchB=on  SwitchC=on  SwitchTimes="[1/60  5/60]"  External=on  BreakerResistance=0.01  SnubberResistance=1e6  SnubberCapacitance=inf  Measurements=None
  VSC_Control : Subsystem
      settings: PortSchema="{\"entries\":[{\"content\":{\"sides\":[{\"content\":{\"connectorIds\":[\"In1\",\"In2\",\"In3\",\"In4\",\"In5\"]},\"type\":\"ConnectorPlacement.EquallySpacedRectSide\",\"uuid\":\"45e52e2a-5d2e-4b01-a357-9d3073978641\"},{\"content\":{\"connectorIds\":[\"Out1\",\"Out2\",\"Out3\"],\"side\":\"RIGHT\"},\"type\":\"ConnectorPlacement.EquallySpacedRectSide\",\"uuid\":\"500a659a-c60e-4c3f-b5c2-04d8fe26286a\"},{\"content\":{\"connectorIds\":[\"In6\",\"In7\"],\"side\":\"TOP\"},\"type\":\"ConnectorPlacement.EquallySpacedRectSide\",\"uuid\":\"e5a9e837-077a-4c9c-b808-725d6018483b\"},{\"content\":{\"connectorIds\":[],\"side\":\"HIDDEN\"},\"type\":\"ConnectorPlacement.EquallySpacedRectSide\",\"uuid\":\"1c877ae8-e0c9-4faf-8b8c-99cd40b797b6\"}]},\"type\":\"ConnectorPlacement.EquallySpacedConnector\",\"uuid\":\"17a691b0-ccba-4cde-88e8-165a3a0c6333\"}],\"packageUris\":[\"http://schema.mathworks.com/mf0/Connector/R2020b\"],\"version\":\"1.0\"}"
  Voltage Measurement : spsVoltageMeasurementLib/Voltage Measurement  PhasorSimulation=off  OutputType=Complex  PSBequivalent=0
  a : PMIOPort  Side=Right
  b : PMIOPort  Port=2  Side=Right
  c : PMIOPort  Port=3  Side=Right
  PV_m : Outport
  tag scope: Painel_m=global
  wires:
  [I_PV] -> Product1/1
  PV Array/1 -> [Painel_m]
  Subsystem/1(Iabc) -> [Iabc_PV]
  [Freq] -> APC_algorithm/1(Freq_m)
  [PV_mode] -> APC_algorithm/3(Enable)
  VSC_Control/1(Uref) -> Product/2
  Product1/1 -> Gain/1
  [V_PV] -> Product1/2
  [V_DC_ref] -> VSC_Control/7(Vdc_ref)
  VSC_Control/2(Freq) -> [Freq]
  Rate Limiter/1 -> PV Array/1
  Iq_ref1/1 -> VSC_Control/4(Iq_ref)
  [Iabc_PV] -> VSC_Control/2(Iabc)
  Gain/1 -> Mean/1
  Bus Selector/1 -> [I_PV]  "<I_PV>"
  [PV_mode] -> VSC_Control/6(PV_mode)
  [Vabc_grid] -> VSC_Control/1(Vabc)
  Voltage Measurement/1 -> [Vdc]
  Product/1 -> Three Phase Converter1/1
  [Vdc] -> VSC_Control/3(Vdc_mes)
  Grid1/1 -> [Vabc_grid]
  [Painel_m] -> Bus Selector/1
  APC_algorithm/1(Vdc_ref) -> [V_DC_ref]
  [Fault] -> APC_algorithm/4(Fault)
  Constant7/1 -> APC_algorithm/2(Freq_ref)
  Mean/1 -> [P_PV], Display2/1
  VSC_Control/3(P_PV) -> Terminator1/1
  Bus Selector/2 -> [V_PV]  "<V_PV>"
  Irra/1 -> Rate Limiter/1
  TempC/1 -> PV Array/2
  [Painel_m] -> VSC_Control/5(Painel_m)
  Grid1/2 -> [Iabc_grid]
  PV_mode/1 -> [PV_mode]
  [Iabc_PV] -> Subsystem1/1(Iabc)
  [Iabc_grid] -> Subsystem1/2(In2)
  [Vdc] -> Subsystem1/3(Vdc)  "Vdc"
  [P_PV] -> Subsystem1/4(P_PV)  "P_PV"
  [Freq] -> Subsystem1/5(Freq)  "Freq"
  Subsystem1/1(Out1) -> PV_m/1
  BRK/1 -> [BRK]
  [BRK] -> Three-Phase Breaker/1
  [BRK] -> Product/1
  connections:
  Subsystem/RConn1 -- L/LConn1
  L1/LConn3 -- SSN Interface Block (3ph)/RConn3
  L/RConn1 -- SSN Interface Block (3ph)/LConn1
  L4/RConn1 -- L4/RConn3 -- Ground/LConn1 -- L4/RConn2
  a/RConn1 -- Grid1/RConn1
  Carga/RConn1 -- Three-Phase Series RLC Load/LConn3
  L1/LConn1 -- SSN Interface Block (3ph)/RConn1
  Three Phase Converter1/RConn1 -- Series RLC Branch/LConn1 -- PV Array/RConn1 -- Voltage Measurement/LConn1
  L1/RConn3 -- L4/LConn3 -- 220 kVA 227V / 440V/RConn3
  L1/RConn2 -- L4/LConn2 -- 220 kVA 227V / 440V/RConn2
  SSN Interface Block (3ph)/LConn2 -- L/RConn2
  Subsystem/LConn1 -- Three Phase Converter1/LConn1
  L1/RConn1 -- 220 kVA 227V / 440V/RConn1 -- L4/LConn1
  Carga/RConn2 -- Three-Phase Series RLC Load/LConn2
  Voltage Measurement/LConn2 -- Three Phase Converter1/RConn2 -- PV Array/RConn2 -- Series RLC Branch/RConn1
  Subsystem/RConn2 -- L/LConn2
  Subsystem/LConn3 -- Three Phase Converter1/LConn3
  Three Phase Converter1/LConn2 -- Subsystem/LConn2
  SSN Interface Block (3ph)/LConn3 -- L/RConn3
  Subsystem/RConn3 -- L/LConn3
  Carga/RConn3 -- Three-Phase Series RLC Load/LConn1
  L1/LConn2 -- SSN Interface Block (3ph)/RConn2
  b/RConn1 -- Grid1/RConn2
  c/RConn1 -- Grid1/RConn3
  Three-Phase Breaker/LConn1 -- 220 kVA 227V / 440V/LConn1
  Three-Phase Breaker/LConn2 -- 220 kVA 227V / 440V/LConn2
  Three-Phase Breaker/LConn3 -- 220 kVA 227V / 440V/LConn3
  Three-Phase Breaker/RConn1 -- Grid1/LConn1
  Three-Phase Breaker/RConn2 -- Grid1/LConn2
  Three-Phase Breaker/RConn3 -- Grid1/LConn3
